simulink model "taller_reto"  (R2025b)
settings: Solver=VariableStepAuto  StartTime=0.0  StopTime=10.0  RelTol=1e-3
settings Model: Creator=DELL  LastModifiedBy=Juan Diego Salinas

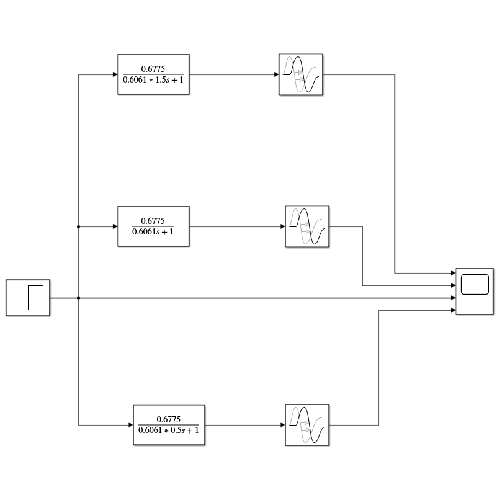
[thumbnail: Simulink's stored preview of the top-level diagram]
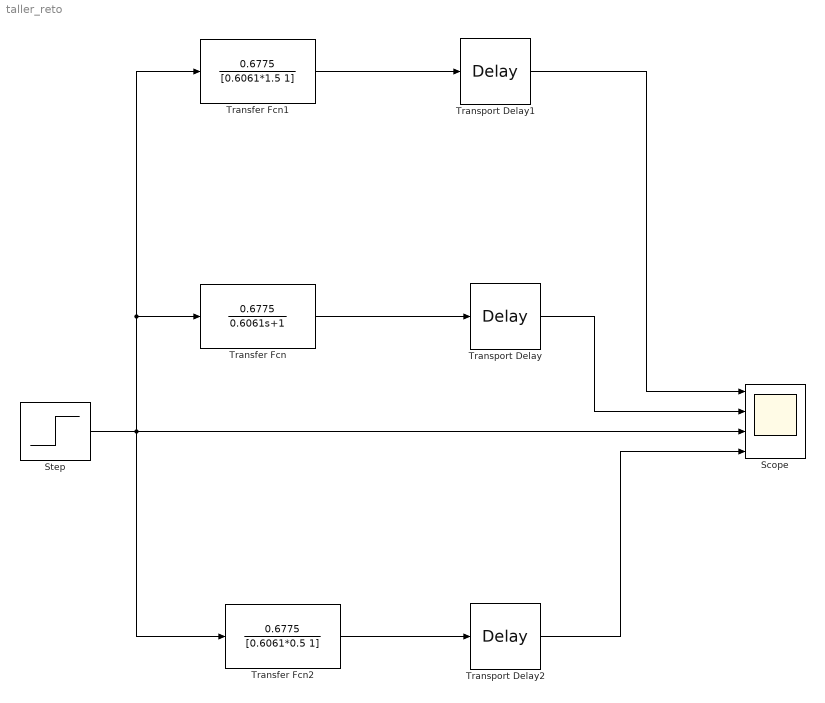
== system taller_reto ==
  Scope : Scope  NumInputPorts=4
      settings: ActiveDisplayYMinimum=-0.18749999999999994  ActiveDisplayYMaximum=1.6875
  Step : Step  After=1.5  SampleTime=0
  Transfer Fcn : TransferFcn  Numerator=[0.6775]  Denominator=[0.6061 1]
  Transfer Fcn1 : TransferFcn  Numerator=[0.6775]  Denominator=[0.6061*1.5 1]
  Transfer Fcn2 : TransferFcn  Numerator=[0.6775]  Denominator=[0.6061*0.5 1]
  Transport Delay : TransportDelay  DelayTime=0.1
  Transport Delay1 : TransportDelay  DelayTime=0.1
  Transport Delay2 : TransportDelay  DelayTime=0.1
  wires:
  Transfer Fcn/1 -> Transport Delay/1
  Transport Delay1/1 -> Scope/1
  Transfer Fcn1/1 -> Transport Delay1/1
  Transport Delay2/1 -> Scope/4
  Step/1 -> Transfer Fcn2/1, Transfer Fcn1/1, Transfer Fcn/1, Scope/3
  Transfer Fcn2/1 -> Transport Delay2/1
  Transport Delay/1 -> Scope/2
